simulink model "Ecotron"  (R2019b)
settings: Solver=FixedStepAuto  StartTime=0.0  StopTime=1  FixedStep=0.001  RelTol=1e-3  EnableMultiTasking=on
InitFcn:
  | EcoCoder_PreCheckLic();
libraries: CoderSF_BSW_Libs x228, SF_CanService_Libs x49, simulink x33, dspstat3 x6
(part 3 of 6)

== system Ecotron/Input/PC/FrontWheelCommands ==
  Bus Creator : BusCreator  Inputs=3
  Bus Creator1 : BusCreator  Inputs=4  OutDataTypeStr=Bus: Msg
      settings: InheritFromInputs=off
  Read CAN Message : SF_CanService_Libs/Read CAN Message  typeCAN=Connected  channel=CAN_D  mEn=off  msgInfo=LeoDrive_vw_GOLF  msgItermStore=FrontWheelCommands  msgIterm=FrontWheelCommands  valid=on  stale=on  motoBit=off  setSignalName=on  flgCustomMonitorVariableRules=on  defineSignalName=off  prefixSignal='PC_'  flgValTest=off  flgNoFixed=on  tSample=Task_L1ms  modeCode=Parameterless
  Subsystem1 : Subsystem
  Write and Read Measurement : CoderSF_BSW_Libs/Calibration & Measurement/Write and Read Measurement  variable_name=PC_SetFrontWheelAngle  variable_value=0  variable_type=single  numD=1  unitStr=""  descStr=""
      settings: AttributesFormatString=type:%<variable_type> Dimensions:%<numD>  SourceProductName=EcoCoder Blocks
  Write and Read Measurement1 : CoderSF_BSW_Libs/Calibration & Measurement/Write and Read Measurement  variable_name=PC_SetFrontWheelAngel_Rate  variable_value=0  variable_type=single  numD=1  unitStr=""  descStr=""
      settings: AttributesFormatString=type:%<variable_type> Dimensions:%<numD>  SourceProductName=EcoCoder Blocks
  Out2 : Outport
  wires:
  Read CAN Message/1 -> Subsystem1/1("Available_in ")
  Bus Creator/1 -> Out2/1
  Read CAN Message/4 -> Write and Read Measurement1/1  "PC_setFront_wheel_angle_rate"
  Subsystem1/2(Cnt) -> Bus Creator1/2  "Cnt"
  Read CAN Message/2 -> Subsystem1/2(Msg_cnt)
  Subsystem1/3(Timeout_Err) -> Bus Creator1/3  "Timeout"
  Read CAN Message/3 -> Write and Read Measurement/1  "PC_setFront_wheel_angle"
  Subsystem1/4(Msg_Freq) -> Bus Creator1/4  "MsgFreq"
  Subsystem1/1("Available ") -> Bus Creator1/1  "Available"
  Write and Read Measurement/1 -> Bus Creator/2  "PC_SetFrontWheelAngle"
  Write and Read Measurement1/1 -> Bus Creator/3  "PC_SetFrontWheelAngel_Rate"
  Bus Creator1/1 -> Bus Creator/1  "Msg"

== system Ecotron/Input/PC/LongitudinalCommands ==
  " Override Probe" : CoderSF_BSW_Libs/Calibration & Measurement/ Override Probe  variableName=SetACC  variableValue=0  overrideValue=0  variableDataType=single  variableMin=[]  variableMax=[]  variableUnitStr=""  variableDescStr=""
  Bus Creator : BusCreator  Inputs=3
  Bus Creator1 : BusCreator  Inputs=4  OutDataTypeStr=Bus: Msg
      settings: InheritFromInputs=off
  Read CAN Message : SF_CanService_Libs/Read CAN Message  typeCAN=Connected  channel=CAN_D  mEn=off  msgInfo=LeoDrive_vw_GOLF  msgItermStore=LongitudinalCommandsV1  msgIterm=LongitudinalCommandsV1  valid=on  stale=on  motoBit=off  setSignalName=on  flgCustomMonitorVariableRules=on  defineSignalName=off  prefixSignal='PC_'  flgValTest=off  flgNoFixed=on  tSample=Task_L1ms  modeCode=Parameterless
  Subsystem1 : Subsystem
  Write and Read Measurement : CoderSF_BSW_Libs/Calibration & Measurement/Write and Read Measurement  variable_name=PC_SetLongAcc  variable_value=0  variable_type=single  numD=1  unitStr=""  descStr=""
      settings: AttributesFormatString=type:%<variable_type> Dimensions:%<numD>  SourceProductName=EcoCoder Blocks
  Write and Read Measurement1 : CoderSF_BSW_Libs/Calibration & Measurement/Write and Read Measurement  variable_name=PC_SetLimitVel  variable_value=0  variable_type=single  numD=1  unitStr=""  descStr=""
      settings: AttributesFormatString=type:%<variable_type> Dimensions:%<numD>  SourceProductName=EcoCoder Blocks
  Out2 : Outport
  wires:
  Subsystem1/1("Available ") -> Bus Creator1/1  "Available"
  Subsystem1/4(Msg_Freq) -> Bus Creator1/4  "MsgFreq"
  Subsystem1/3(Timeout_Err) -> Bus Creator1/3  "Timeout"
  Read CAN Message/2 -> Subsystem1/2(Msg_cnt)
  Subsystem1/2(Cnt) -> Bus Creator1/2  "Cnt"
  Read CAN Message/4 -> Write and Read Measurement1/1  "PC_setLimit_velocity"
  Bus Creator/1 -> Out2/1
  Read CAN Message/1 -> Subsystem1/1("Available_in ")
  Read CAN Message/3 -> Write and Read Measurement/1  "PC_setLong_accel"
  Write and Read Measurement/1 -> " Override Probe"/1  "PC_SetLongAcc"
  Write and Read Measurement1/1 -> Bus Creator/3  "PC_SetLimitVel"
  Bus Creator1/1 -> Bus Creator/1  "Msg"
  " Override Probe"/1 -> Bus Creator/2  "SetACCOvrMsr"

== system Ecotron/Input/PC/LongitudinalCommandsV2 ==
  Bus Creator : BusCreator  Inputs=3
  Bus Creator1 : BusCreator  Inputs=4  OutDataTypeStr=Bus: Msg
      settings: InheritFromInputs=off
  Read CAN Message : SF_CanService_Libs/Read CAN Message  typeCAN=Connected  channel=CAN_D  mEn=off  msgInfo=LeoDrive_vw_GOLF  msgItermStore=LongitudinalCommandsV2  msgIterm=LongitudinalCommandsV2  valid=on  stale=on  motoBit=off  setSignalName=on  flgCustomMonitorVariableRules=on  defineSignalName=off  prefixSignal='PC_'  flgValTest=off  flgNoFixed=on  tSample=Task_L1ms  modeCode=Parameterless
  Subsystem1 : Subsystem
  Write and Read Measurement : CoderSF_BSW_Libs/Calibration & Measurement/Write and Read Measurement  variable_name=PC_SetGasPos  variable_value=0  variable_type=single  numD=1  unitStr=""  descStr=""
      settings: AttributesFormatString=type:%<variable_type> Dimensions:%<numD>  SourceProductName=EcoCoder Blocks
  Write and Read Measurement1 : CoderSF_BSW_Libs/Calibration & Measurement/Write and Read Measurement  variable_name=PC_SetBrakePos  variable_value=0  variable_type=single  numD=1  unitStr=""  descStr=""
      settings: AttributesFormatString=type:%<variable_type> Dimensions:%<numD>  SourceProductName=EcoCoder Blocks
  Out2 : Outport
  wires:
  Read CAN Message/1 -> Subsystem1/1("Available_in ")
  Bus Creator/1 -> Out2/1
  Read CAN Message/4 -> Write and Read Measurement1/1  "PC_setBrake_pedal_pos"
  Subsystem1/2(Cnt) -> Bus Creator1/2  "Cnt"
  Read CAN Message/2 -> Subsystem1/2(Msg_cnt)
  Subsystem1/3(Timeout_Err) -> Bus Creator1/3  "Timeout"
  Read CAN Message/3 -> Write and Read Measurement/1  "PC_setGas_pedal_pos"
  Subsystem1/4(Msg_Freq) -> Bus Creator1/4  "MsgFreq"
  Subsystem1/1("Available ") -> Bus Creator1/1  "Available"
  Write and Read Measurement/1 -> Bus Creator/2  "PC_SetGasPos"
  Write and Read Measurement1/1 -> Bus Creator/3  "PC_SetBrakePos"
  Bus Creator1/1 -> Bus Creator/1  "Msg"

== system Ecotron/Input/PC/Vehicle_Commands ==
  Bus Creator : BusCreator  Inputs=8
  Bus Creator1 : BusCreator  Inputs=4  OutDataTypeStr=Bus: Msg
      settings: InheritFromInputs=off
  Read CAN Message : SF_CanService_Libs/Read CAN Message  typeCAN=Connected  channel=CAN_D  mEn=off  msgInfo=LeoDrive_vw_GOLF  msgItermStore=VehicleCommands  msgIterm=VehicleCommands  valid=on  stale=on  motoBit=off  setSignalName=on  flgCustomMonitorVariableRules=on  defineSignalName=off  prefixSignal='PC_'  flgValTest=off  flgNoFixed=on  tSample=Task_L1ms  modeCode=Parameterless
  Subsystem1 : Subsystem
  Terminator1 : Terminator
  Write and Read Measurement : CoderSF_BSW_Libs/Calibration & Measurement/Write and Read Measurement  variable_name=PC_blinker  variable_value=0  variable_type=uint8  numD=1  unitStr=""  descStr=""
      settings: AttributesFormatString=type:%<variable_type> Dimensions:%<numD>  SourceProductName=EcoCoder Blocks
  Write and Read Measurement1 : CoderSF_BSW_Libs/Calibration & Measurement/Write and Read Measurement  variable_name=PC_headlight  variable_value=0  variable_type=uint8  numD=1  unitStr=""  descStr=""
      settings: AttributesFormatString=type:%<variable_type> Dimensions:%<numD>  SourceProductName=EcoCoder Blocks
  Write and Read Measurement2 : CoderSF_BSW_Libs/Calibration & Measurement/Write and Read Measurement  variable_name=PC_wiper  variable_value=0  variable_type=uint8  numD=1  unitStr=""  descStr=""
      settings: AttributesFormatString=type:%<variable_type> Dimensions:%<numD>  SourceProductName=EcoCoder Blocks
  Write and Read Measurement3 : CoderSF_BSW_Libs/Calibration & Measurement/Write and Read Measurement  variable_name=PC_gear  variable_value=0  variable_type=uint8  numD=1  unitStr=""  descStr=""
      settings: AttributesFormatString=type:%<variable_type> Dimensions:%<numD>  SourceProductName=EcoCoder Blocks
  Write and Read Measurement4 : CoderSF_BSW_Libs/Calibration & Measurement/Write and Read Measurement  variable_name=PC_mode  variable_value=0  variable_type=uint8  numD=1  unitStr=""  descStr=""
      settings: AttributesFormatString=type:%<variable_type> Dimensions:%<numD>  SourceProductName=EcoCoder Blocks
  Write and Read Measurement5 : CoderSF_BSW_Libs/Calibration & Measurement/Write and Read Measurement  variable_name=PC_handBrake  variable_value=0  variable_type=uint8  numD=1  unitStr=""  descStr=""
      settings: AttributesFormatString=type:%<variable_type> Dimensions:%<numD>  SourceProductName=EcoCoder Blocks
  Write and Read Measurement6 : CoderSF_BSW_Libs/Calibration & Measurement/Write and Read Measurement  variable_name=PC_LongMode  variable_value=0  variable_type=uint8  numD=1  unitStr=""  descStr=""
      settings: AttributesFormatString=type:%<variable_type> Dimensions:%<numD>  SourceProductName=EcoCoder Blocks
  Out1 : Outport
  wires:
  Subsystem1/2(Cnt) -> Bus Creator1/2  "Cnt"
  Read CAN Message/2 -> Subsystem1/2(Msg_cnt)
  Subsystem1/4(Msg_Freq) -> Bus Creator1/4  "MsgFreq"
  Read CAN Message/7 -> Write and Read Measurement4/1  "PC_mode"
  Bus Creator/1 -> Out1/1
  Subsystem1/3(Timeout_Err) -> Bus Creator1/3  "Timeout"
  Read CAN Message/8 -> Write and Read Measurement5/1  "PC_handBrake"
  Subsystem1/1("Available ") -> Bus Creator1/1  "Available"
  Read CAN Message/3 -> Write and Read Measurement/1  "PC_blinker"
  Read CAN Message/5 -> Write and Read Measurement2/1  "PC_wiper"
  Read CAN Message/1 -> Subsystem1/1("Available_in ")
  Read CAN Message/4 -> Write and Read Measurement1/1  "PC_headlgiht"
  Read CAN Message/10 -> Write and Read Measurement6/1  "PC_LongMode"
  Read CAN Message/9 -> Terminator1/1  "PC_horn"
  Write and Read Measurement/1 -> Bus Creator/2  "PC_blinker"
  Write and Read Measurement1/1 -> Bus Creator/3  "PC_headlight"
  Write and Read Measurement2/1 -> Bus Creator/4  "PC_wiper"
  Read CAN Message/6 -> Write and Read Measurement3/1  "PC_gear"
  Write and Read Measurement3/1 -> Bus Creator/5  "PC_gear"
  Write and Read Measurement4/1 -> Bus Creator/6  "PC_mode"
  Write and Read Measurement5/1 -> Bus Creator/7  "PC_handBrake"
  Bus Creator1/1 -> Bus Creator/1  "Msg"
  Write and Read Measurement6/1 -> Bus Creator/8  "PC_LongMode"

== system Ecotron/Main /Err Handler/Check Brake Err ==
  In1 : Inport
  Bus Creator : BusCreator  Inputs=2
  Bus Selector : BusSelector  OutputSignals=By-wire.RBF_Brake.EPAS_Msg3.BBW_UnderVoltage,By-wire.RBF_Brake.EPAS_Msg3.BBW_OverCurrent,By-wire.RBF_Brake.EPAS_Msg1.Msg.timeout,By-wire.RBF_Brake.EPAS_Msg2.Msg.timeout,By-wire.RBF_Brake.EPAS_Msg3.Msg.timeout
  OR : Logic  Operator=OR  IconShape=distinctive  AllPortsSameDT=off  OutDataTypeStr=boolean
  OR1 : Logic  Operator=OR  Inputs=3  IconShape=distinctive  AllPortsSameDT=off  OutDataTypeStr=boolean
  Out1 : Outport
  wires:
  In1/1 -> Bus Selector/1
  Bus Selector/1 -> OR/1  "<BBW_UnderVoltage>"
  Bus Selector/2 -> OR/2  "<BBW_OverCurrent>"
  Bus Selector/3 -> OR1/1  "<timeout>"
  Bus Selector/4 -> OR1/2  "<timeout>"
  Bus Selector/5 -> OR1/3  "<timeout>"
  OR/1 -> Bus Creator/1  "Brake_SystemErr"
  OR1/1 -> Bus Creator/2  "Brake_HeartBeatErr"
  Bus Creator/1 -> Out1/1

== system Ecotron/Main /Err Handler/Check EPAS Err ==
  In1 : Inport
  Bus Creator : BusCreator  Inputs=2
  Bus Selector : BusSelector  OutputSignals=By-wire.EPAS.EPAS_Msg3.EPAS_UnderVoltage,By-wire.EPAS.EPAS_Msg3.EPAS_OverCurrent,By-wire.EPAS.EPAS_Msg1.Msg.timeout,By-wire.EPAS.EPAS_Msg2.Msg.timeout,By-wire.EPAS.EPAS_Msg3.Msg.timeout
  OR : Logic  Operator=OR  IconShape=distinctive  AllPortsSameDT=off  OutDataTypeStr=boolean
  OR1 : Logic  Operator=OR  Inputs=3  IconShape=distinctive  AllPortsSameDT=off  OutDataTypeStr=boolean
  Epas_Errors : Outport
  wires:
  In1/1 -> Bus Selector/1
  Bus Selector/1 -> OR/1  "<EPAS_UnderVoltage>"
  Bus Selector/2 -> OR/2  "<EPAS_OverCurrent>"
  OR/1 -> Bus Creator/1  "EPAS_SystemErr"
  Bus Selector/3 -> OR1/1  "<timeout>"
  Bus Selector/4 -> OR1/2  "<timeout>"
  Bus Selector/5 -> OR1/3  "<timeout>"
  OR1/1 -> Bus Creator/2  "EPAS_HeartbeatErr"
  Bus Creator/1 -> Epas_Errors/1

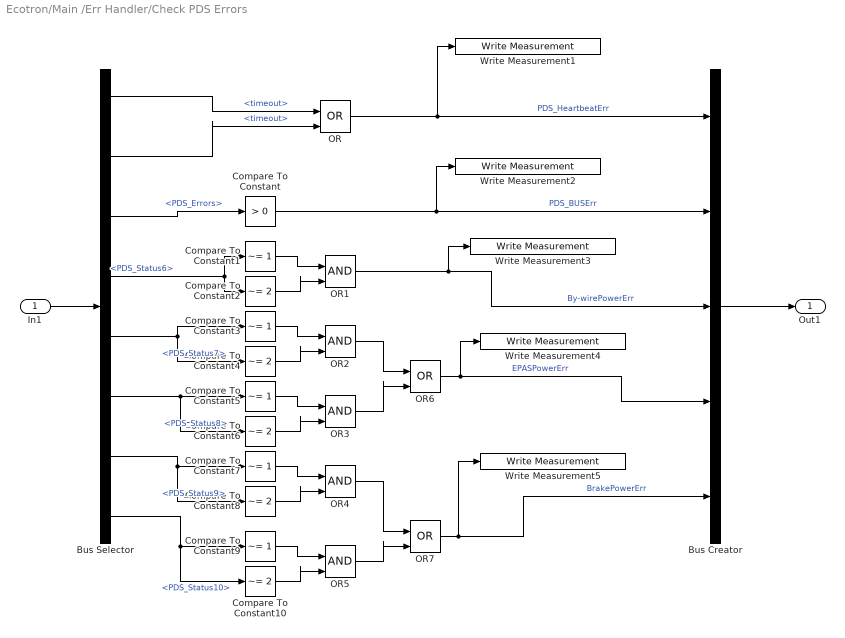
== system Ecotron/Main /Err Handler/Check PDS Errors ==
  In1 : Inport
  Bus Creator : BusCreator  Inputs=5
  Bus Selector : BusSelector  OutputSignals=By-wire.PDS.Status.Msg.timeout,By-wire.PDS.Status2.Msg.timeout,By-wire.PDS.Status.PDS_Errors,By-wire.PDS.Status.PDS_Status6,By-wire.PDS.Status.PDS_Status7,By-wire.PDS.Status.PDS_Status8,By-wire.PDS.Status.PDS_Status9,By-wire.PDS.Status.PDS_Status10
  Compare To Constant : simulink/Logic and Bit Operations/Compare To Constant  relop=>  const=0  OutDataTypeStr=boolean
  Compare To Constant{1,3,5,7,9} (5 alike) : simulink/Logic and Bit Operations/Compare To Constant  relop=~=  const=1  OutDataTypeStr=boolean
  Compare To Constant{2,4,6,8,10} (5 alike) : simulink/Logic and Bit Operations/Compare To Constant  relop=~=  const=2  OutDataTypeStr=boolean
  OR : Logic  Operator=OR  IconShape=distinctive  AllPortsSameDT=off  OutDataTypeStr=boolean
  OR{1..5} (5 alike) : Logic  IconShape=distinctive  AllPortsSameDT=off  OutDataTypeStr=boolean
  OR6 : Logic  Operator=OR  IconShape=distinctive  AllPortsSameDT=off  OutDataTypeStr=boolean
  OR7 : Logic  Operator=OR  IconShape=distinctive  AllPortsSameDT=off  OutDataTypeStr=boolean
  Write Measurement1 : CoderSF_BSW_Libs/Calibration & Measurement/Write Measurement  variable_name=Diag_PDS_HeartbeatErr  variable_value=0  variable_type=boolean  numD=1  unitStr=""  descStr=""
      settings: AttributesFormatString=type:%<variable_type> Dimensions:%<numD>  SourceProductName=EcoCoder Blocks
  Write Measurement2 : CoderSF_BSW_Libs/Calibration & Measurement/Write Measurement  variable_name=Diag_PDS_BUSErr  variable_value=0  variable_type=boolean  numD=1  unitStr=""  descStr=""
      settings: AttributesFormatString=type:%<variable_type> Dimensions:%<numD>  SourceProductName=EcoCoder Blocks
  Write Measurement3 : CoderSF_BSW_Libs/Calibration & Measurement/Write Measurement  variable_name=Diag_By_wirePowerErr  variable_value=0  variable_type=boolean  numD=1  unitStr=""  descStr=""
      settings: AttributesFormatString=type:%<variable_type> Dimensions:%<numD>  SourceProductName=EcoCoder Blocks
  Write Measurement4 : CoderSF_BSW_Libs/Calibration & Measurement/Write Measurement  variable_name=Diag_EPASPowerErr  variable_value=0  variable_type=boolean  numD=1  unitStr=""  descStr=""
      settings: AttributesFormatString=type:%<variable_type> Dimensions:%<numD>  SourceProductName=EcoCoder Blocks
  Write Measurement5 : CoderSF_BSW_Libs/Calibration & Measurement/Write Measurement  variable_name=Diag_BrakePowerErr  variable_value=0  variable_type=boolean  numD=1  unitStr=""  descStr=""
      settings: AttributesFormatString=type:%<variable_type> Dimensions:%<numD>  SourceProductName=EcoCoder Blocks
  Out1 : Outport
  wires:
  In1/1 -> Bus Selector/1
  Bus Selector/1 -> OR/1  "<timeout>"
  Bus Selector/2 -> OR/2  "<timeout>"
  Bus Selector/3 -> Compare To Constant/1  "<PDS_Errors>"
  Bus Selector/4 -> Compare To Constant2/1, Compare To Constant1/1  "<PDS_Status6>"
  Compare To Constant1/1 -> OR1/1
  Compare To Constant2/1 -> OR1/2
  Compare To Constant4/1 -> OR2/2
  Compare To Constant3/1 -> OR2/1
  Compare To Constant5/1 -> OR3/1
  Compare To Constant6/1 -> OR3/2
  Compare To Constant8/1 -> OR4/2
  Compare To Constant7/1 -> OR4/1
  Compare To Constant9/1 -> OR5/1
  Compare To Constant10/1 -> OR5/2
  Bus Selector/5 -> Compare To Constant3/1, Compare To Constant4/1  "<PDS_Status7>"
  Bus Selector/6 -> Compare To Constant6/1, Compare To Constant5/1  "<PDS_Status8>"
  Bus Selector/7 -> Compare To Constant8/1, Compare To Constant7/1  "<PDS_Status9>"
  Bus Selector/8 -> Compare To Constant10/1, Compare To Constant9/1  "<PDS_Status10>"
  OR/1 -> Write Measurement1/1, Bus Creator/1  "PDS_HeartbeatErr"
  Compare To Constant/1 -> Write Measurement2/1, Bus Creator/2  "PDS_BUSErr"
  OR1/1 -> Write Measurement3/1, Bus Creator/3  "By-wirePowerErr"
  OR2/1 -> OR6/1
  OR3/1 -> OR6/2
  OR6/1 -> Write Measurement4/1, Bus Creator/4  "EPASPowerErr"
  OR4/1 -> OR7/1
  OR5/1 -> OR7/2
  OR7/1 -> Write Measurement5/1, Bus Creator/5  "BrakePowerErr"
  Bus Creator/1 -> Out1/1

== system Ecotron/Main /Err Handler/Check Throttle ECU Errors ==
  In1 : Inport
  Bus Creator : BusCreator  Inputs=2
  Bus Selector : BusSelector  OutputSignals=By-wire.Throttle.THROTTLE_CurrentPedalPos,By-wire.Throttle.Msg.timeout
  Compare To Constant : simulink/Logic and Bit Operations/Compare To Constant  relop=>  const=5  OutDataTypeStr=boolean
  Compare To Constant1 : simulink/Logic and Bit Operations/Compare To Constant  relop=>  const=0  OutDataTypeStr=boolean
  Out1 : Outport
  wires:
  In1/1 -> Bus Selector/1
  Bus Selector/1 -> Compare To Constant/1  "<THROTTLE_CurrentPedalPos>"
  Compare To Constant/1 -> Bus Creator/1  "GasPedalintervention"
  Bus Creator/1 -> Out1/1
  Bus Selector/2 -> Compare To Constant1/1  "<timeout>"
  Compare To Constant1/1 -> Bus Creator/2  "Throttle_ECU_HeartbeatErr"

== system Ecotron/Main /Err Handler/MotorStatus ==
  In1 : Inport
  Bus Creator : BusCreator  Inputs=2
  Bus Selector : BusSelector  OutputSignals=vehicle.MotorRotationSpeed.GOLF_MotorRPM,vehicle.Kontak.GOLF_StartStop,vehicle.Kontak.GOLF_KL75
  Compare To Constant : simulink/Logic and Bit Operations/Compare To Constant  relop=>  const=0  OutDataTypeStr=boolean
  Delay : Delay  DelayLength=10  SampleTime=0.1
  OR : Logic  Operator=OR  Inputs=3  IconShape=distinctive  AllPortsSameDT=off  OutDataTypeStr=boolean
  OR1 : Logic  Operator=OR  IconShape=distinctive  AllPortsSameDT=off  OutDataTypeStr=boolean
  RPM : Constant  Value=600  OutDataTypeStr=single
  Relational Operator : RelationalOperator  Operator=<=  OutDataTypeStr=boolean  RndMeth=Simplest
  Write Measurement : CoderSF_BSW_Libs/Calibration & Measurement/Write Measurement  variable_name=Diag_isMotorrunning  variable_value=0  variable_type=boolean  numD=1  unitStr=""  descStr=""
      settings: AttributesFormatString=type:%<variable_type> Dimensions:%<numD>  SourceProductName=EcoCoder Blocks
  Write Measurement1 : CoderSF_BSW_Libs/Calibration & Measurement/Write Measurement  variable_name=Diag_KL75  variable_value=0  variable_type=boolean  numD=1  unitStr=""  descStr=""
      settings: AttributesFormatString=type:%<variable_type> Dimensions:%<numD>  SourceProductName=EcoCoder Blocks
  Motor : Outport
  wires:
  In1/1 -> Bus Selector/1
  Bus Selector/1 -> Relational Operator/2  "<GOLF_MotorRPM>"
  Bus Selector/3 -> Delay/1, OR/2  "<GOLF_KL75>"
  RPM/1 -> Relational Operator/1
  Relational Operator/1 -> OR1/1
  Delay/1 -> OR/3
  OR/1 -> Bus Creator/2, Write Measurement1/1  "Kl75"
  Bus Creator/1 -> Motor/1
  Bus Selector/2 -> Compare To Constant/1  "<GOLF_StartStop>"
  Compare To Constant/1 -> OR1/2
  OR1/1 -> OR/1, Write Measurement/1, Bus Creator/1  "isMotorRunning"

== system Ecotron/Main /Err Handler/Subsystem ==
  In1 : Inport
  AND : Logic  IconShape=distinctive  AllPortsSameDT=off  OutDataTypeStr=boolean
  Bus Selector : BusSelector  OutputSignals=PC.VehicleCMD.Msg.timeout,PC.FrontWheelCMD.Msg.timeout,PC.LongCMD.Msg.timeout,PC.LongV2CMD.Msg.timeout
  OR : Logic  Operator=OR  Inputs=3  IconShape=distinctive  AllPortsSameDT=off  OutDataTypeStr=boolean
  Out1 : Outport
  wires:
  In1/1 -> Bus Selector/1
  Bus Selector/1 -> OR/1  "<timeout>"
  Bus Selector/2 -> OR/2  "<timeout>"
  OR/1 -> Out1/1  "PC_timeout"
  AND/1 -> OR/3
  Bus Selector/3 -> AND/1  "<timeout>"
  Bus Selector/4 -> AND/2  "<timeout>"

== system Ecotron/Main /Gear/Gear_Control ==
  GOLF_CurrentGear : Inport
  Available : Inport  Port=2
  "Set_gear " : Inport  Port=3  OutDataTypeStr=uint8
  Enable : Inport  Port=4
  ParkEnable : Inport  Port=5
  " Override Probe" : CoderSF_BSW_Libs/Calibration & Measurement/ Override Probe  variableName=Set_Gear  variableValue=1  overrideValue=0  variableDataType=uint8  variableMin=[]  variableMax=[]  variableUnitStr=""  variableDescStr=""
      settings: SourceProductName=EcoCoder Blocks
  AND : Logic  IconShape=distinctive  AllPortsSameDT=off  OutDataTypeStr=boolean
  Bus Creator : BusCreator  Inputs=7
  Chart : Stateflow chart  BlockKeywords=__PRM__SERIALIZED__DATA__:Stateflow Chart,Stateflow Diagram  TreatAsAtomicUnit=on
  Chart1 : Stateflow chart  BlockKeywords=__PRM__SERIALIZED__DATA__:Stateflow Chart,Stateflow Diagram  TreatAsAtomicUnit=on
  Data Type Conversion2 : DataTypeConversion  OutDataTypeStr=single
  GOLF_CurrentGear1 : InportShadow
  Read Calibration16 : CoderSF_BSW_Libs/Calibration & Measurement/Read Calibration  variable_name=repeat  variable_value=5  variable_type=single  variable_min=[]  variable_max=[]  unitStr=""  descStr=""
      settings: AttributesFormatString=value:%<variable_value> type:%<variable_type> max:%<variable_max> Min:%<variable_min>  SourceProductName=EcoCoder Blocks
  Read Calibration17 : CoderSF_BSW_Libs/Calibration & Measurement/Read Calibration  variable_name=interval  variable_value=0  variable_type=single  variable_min=[]  variable_max=[]  unitStr=""  descStr=""
      settings: AttributesFormatString=value:%<variable_value> type:%<variable_type> max:%<variable_max> Min:%<variable_min>  SourceProductName=EcoCoder Blocks
  Read Calibration18 : CoderSF_BSW_Libs/Calibration & Measurement/Read Calibration  variable_name=interval2  variable_value=0  variable_type=single  variable_min=[]  variable_max=[]  unitStr=""  descStr=""
      settings: AttributesFormatString=value:%<variable_value> type:%<variable_type> max:%<variable_max> Min:%<variable_min>  SourceProductName=EcoCoder Blocks
  Read Calibration19 : CoderSF_BSW_Libs/Calibration & Measurement/Read Calibration  variable_name=Delay  variable_value=0  variable_type=single  variable_min=[]  variable_max=[]  unitStr=""  descStr=""
      settings: AttributesFormatString=value:%<variable_value> type:%<variable_type> max:%<variable_max> Min:%<variable_min>  SourceProductName=EcoCoder Blocks
  Write Measurement2 : CoderSF_BSW_Libs/Calibration & Measurement/Write Measurement  variable_name=gear_cnt  variable_value=0  variable_type=single  numD=1  unitStr=""  descStr=""
      settings: AttributesFormatString=type:%<variable_type> Dimensions:%<numD>  SourceProductName=EcoCoder Blocks
  Gear_Trigger : Outport
  wires:
  Data Type Conversion2/1 -> Write Measurement2/1
  " Override Probe"/1 -> Chart1/1(SetGear), Chart/2(SetGear)  "Set_GearOvrMsr"
  Available/1 -> Chart1/3(Available)
  Chart1/1(cnt) -> Data Type Conversion2/1
  Read Calibration17/1 -> Chart1/4(interval)
  Read Calibration19/1 -> Chart1/7(delay)
  Read Calibration16/1 -> Chart1/5(msglimit)
  Read Calibration18/1 -> Chart1/6(interval2)
  "Set_gear "/1 -> " Override Probe"/1
  Chart1/2(PtoNTrigger) -> Bus Creator/1  "PtoN"
  Chart1/3(PtoDTrigger) -> Bus Creator/2  "PtoD"
  Chart1/4(DtoNTrigger) -> Bus Creator/3  "DtoN"
  Chart1/5(NtoDTrigger) -> Bus Creator/4  "NtoD"
  Chart1/6(NtoRTrigger) -> Bus Creator/5  "NtoR"
  Chart1/7(RtoNTrigger) -> Bus Creator/6  "RtoN"
  Bus Creator/1 -> Gear_Trigger/1
  Enable/1 -> AND/1, Chart1/8(ENABLE)
  GOLF_CurrentGear/1 -> Chart1/2(CurrentGear)  "GOLF_CurrentGear"
  Chart/1(Parktrigger) -> Bus Creator/7
  GOLF_CurrentGear1/1 -> Chart/1(CurrentGear)  "GOLF_CurrentGear"
  ParkEnable/1 -> AND/2
  AND/1 -> Chart/3(ENABLE)

== system Ecotron/Main /LateralControl/Steering Map ==
  Wheel Rad : Inport
  1-D Lookup Table : Lookup_n-D  NumberOfTableDimensions=1  BreakpointsForDimension1=|  Table=|  InternalRulePriority=Speed  RndMeth=Simplest  InputSameDT=on
      BreakpointsForDimension1=|
      | flip([0.588388039
      | 0.557493058
      | 0.486732906
      | 0.4203094
      | 0.355219971
      | 0.297543446
      | 0.234858963
      | 0.17645621
      | 0.118457225
      | 0.089293954
      | 0.059559667
      | 0.023670812
      | 0.011877895
      | 0.006137322
      | -0.006137322
      | -0.011877895
      | -0.023670812
      | -0.059559667
      | -0.089293954
      | -0.118457225
      | -0.17645621
      | -0.234858963
      | -0.297543446
      | -0.355219971
      | -0.4203094
      | -0.486732906
      | -0.557493058
      | -0.588388039])
      Table=|
      | flip([470
      | 450
      | 400
      | 350
      | 300
      | 250
      | 200
      | 150
      | 100
      | 75
      | 50
      | 20
      | 10
      | 5
      | -5
      | -10
      | -20
      | -50
      | -75
      | -100
      | -150
      | -200
      | -250
      | -300
      | -350
      | -400
      | -450
      | -470
      | ])
  Steering Wheel Degree : Outport
  wires:
  Wheel Rad/1 -> 1-D Lookup Table/1
  1-D Lookup Table/1 -> Steering Wheel Degree/1

== system Ecotron/Main /LongControl /ACC Control ==
  In2 : Inport
  Bus Selector : BusSelector  OutputSignals=input.PC.LongCMD.SetACCOvrMsr,input.vehicle.MotorTorque.GOLF_MotorTorque_filtered,input.vehicle.GearLevel.GOLF_GearLevel,input.vehicle.ACC.GOLF_rxACC
  "Fcalculator " : Subsystem
  Long PID : Subsystem  Commented=on
  StopModeDesicion : Subsystem
  VehicleSpeed : Subsystem
  gas : Outport
  brake : Outport  Port=2
  StopMode : Outport  Port=3
  wires:
  VehicleSpeed/1(m/s) -> StopModeDesicion/1(speed), "Fcalculator "/2(m/s), Long PID/5(speed)
  In2/1 -> Bus Selector/1, "Fcalculator "/1(In1), StopModeDesicion/2(bus), VehicleSpeed/1(In1)
  Bus Selector/1 -> Long PID/1(ACC cmd)  "<SetACCOvrMsr>"
  StopModeDesicion/1(StopModeEnable) -> StopMode/1, "Fcalculator "/3(StopModeEnable), Long PID/6(StopModeEnable)
  Bus Selector/2 -> Long PID/2(MotorTorque)  "<GOLF_MotorTorque_filtered>"
  Bus Selector/3 -> Long PID/3(Gear)  "<GOLF_GearLevel>"
  Bus Selector/4 -> Long PID/4(AccFeedback)  "<GOLF_rxACC>"
  "Fcalculator "/2(Brake Pedal) -> brake/1
  "Fcalculator "/1(Gas Pedal) -> gas/1

== system Ecotron/Main /LongControl /Brake Calib logic ==
  In1 : Inport
  " Override Probe" : CoderSF_BSW_Libs/Calibration & Measurement/ Override Probe  variableName=Brake_CalibCMD  variableValue=0  overrideValue=0  variableDataType=single  variableMin=[]  variableMax=[]  variableUnitStr=""  variableDescStr=""
      settings: SourceProductName=EcoCoder Blocks
  Bus Selector : BusSelector  OutputSignals=Errors.Motor.isMotorRunning,input.vehicle.BrakePedal.GOLF_BrakePedalPos,input.By-wire.RBF_Brake.EPAS_Msg3.BBW_OnCalibration,input.By-wire.RBF_Brake.EPAS_Msg3.BBW_CalibrationErr,input.vehicle.WheelSpeed.GOLF_FLWheelSpeed
  Chart : Stateflow chart  BlockKeywords=__PRM__SERIALIZED__DATA__:Stateflow Chart,Stateflow Diagram  TreatAsAtomicUnit=on
  Out1 : Outport
  wires:
  " Override Probe"/1 -> Out1/1  "Brake_CalibCMDOvrMsr"
  In1/1 -> Bus Selector/1
  Bus Selector/1 -> Chart/1(isMotorRunning)  "<isMotorRunning>"
  Bus Selector/2 -> Chart/2(BrakePedalPos)  "<GOLF_BrakePedalPos>"
  Bus Selector/3 -> Chart/3(BBW_OnCalibration)  "<BBW_OnCalibration>"
  Bus Selector/4 -> Chart/4(BBW_CalibrationErr)  "<BBW_CalibrationErr>"
  Chart/1(Calib_CMD) -> " Override Probe"/1
  Bus Selector/5 -> Chart/5(speed)  "<GOLF_FLWheelSpeed>"

== system Ecotron/Subsystem4/Button cntrl /Subsystem ==
  "Start-Stop " : Inport
  Start_Stop1 : CoderSF_BSW_Libs/Digital I//O/Switch Output  channel=HSO01
      settings: SourceProductName=EcoCoder Blocks
  Start_Stop2 : CoderSF_BSW_Libs/Digital I//O/Switch Output  channel=HSO02
      settings: SourceProductName=EcoCoder Blocks
  Unit Delay : UnitDelay  SampleTime=0.1  HasFrameUpgradeWarning=on
  wires:
  "Start-Stop "/1 -> Start_Stop1/1, Unit Delay/1
  Unit Delay/1 -> Start_Stop2/1

== system Ecotron/Subsystem4/Button cntrl /Subsystem1 ==
  Left_in : Inport
  Right_in : Inport  Port=2
  Hazard_in : Inport  Port=3
  Headligh_in : Inport  Port=4
  Flasher_in : Inport  Port=5
  Mode : Inport  Port=6
  timeout : Inport  Port=7
  AND : Logic  IconShape=distinctive  AllPortsSameDT=off  OutDataTypeStr=boolean
  Compare To Constant : simulink/Logic and Bit Operations/Compare To Constant  relop===  const=1  OutDataTypeStr=boolean
  Compare To Constant1 : simulink/Logic and Bit Operations/Compare To Constant  relop===  const=0  OutDataTypeStr=boolean
  Constant : Constant  Value=0  OutDataTypeStr=boolean
  Switch{,1..4} (5 alike) : Switch  Criteria=u2 > Threshold
  Left_out : Outport
  Right_out : Outport  Port=2
  Hazard_out : Outport  Port=3
  Headlight_out : Outport  Port=4
  Flasher_out : Outport  Port=5
  wires:
  Mode/1 -> Compare To Constant/1
  timeout/1 -> Compare To Constant1/1
  Compare To Constant/1 -> AND/1
  Compare To Constant1/1 -> AND/2
  Left_in/1 -> Switch/1
  Switch/1 -> Left_out/1
  Right_in/1 -> Switch1/1
  Hazard_in/1 -> Switch2/1
  Headligh_in/1 -> Switch3/1
  Flasher_in/1 -> Switch4/1
  AND/1 -> Switch/2, Switch1/2, Switch2/2, Switch3/2, Switch4/2
  Constant/1 -> Switch4/3, Switch3/3, Switch2/3, Switch1/3, Switch/3
  Switch4/1 -> Flasher_out/1
  Switch3/1 -> Headlight_out/1
  Switch2/1 -> Hazard_out/1
  Switch1/1 -> Right_out/1

== system Ecotron/Subsystem4/Button cntrl /Subsystem4 ==
  mode : Inport
  Chart : Stateflow chart  BlockKeywords=__PRM__SERIALIZED__DATA__:Stateflow Chart,Stateflow Diagram  TreatAsAtomicUnit=on
  Falling Edge : CoderSF_BSW_Libs/Application Base Blocks/Falling Edge  InitialCondition=off
      settings: SourceProductName=EcoCoder Blocks
  Read Calibration : CoderSF_BSW_Libs/Calibration & Measurement/Read Calibration  variable_name=Buzz_rising_duration  variable_value=500  variable_type=single  variable_min=[]  variable_max=[]  unitStr=""  descStr=""
      settings: AttributesFormatString=value:%<variable_value> type:%<variable_type> max:%<variable_max> Min:%<variable_min>  SourceProductName=EcoCoder Blocks
  Read Calibration1 : CoderSF_BSW_Libs/Calibration & Measurement/Read Calibration  variable_name=Buzz_falling_duration  variable_value=500  variable_type=single  variable_min=[]  variable_max=[]  unitStr=""  descStr=""
      settings: AttributesFormatString=value:%<variable_value> type:%<variable_type> max:%<variable_max> Min:%<variable_min>  SourceProductName=EcoCoder Blocks
  Read Calibration2 : CoderSF_BSW_Libs/Calibration & Measurement/Read Calibration  variable_name=Buzz_falling_offduration  variable_value=250  variable_type=single  variable_min=[]  variable_max=[]  unitStr=""  descStr=""
      settings: AttributesFormatString=value:%<variable_value> type:%<variable_type> max:%<variable_max> Min:%<variable_min>  SourceProductName=EcoCoder Blocks
  Rising Edge : CoderSF_BSW_Libs/Application Base Blocks/Rising Edge  InitialCondition=on
      settings: SourceProductName=EcoCoder Blocks
  out : Outport
  wires:
  mode/1 -> Falling Edge/1, Rising Edge/1
  Rising Edge/1 -> Chart/1(risingedge)
  Falling Edge/1 -> Chart/2(fallingedge)
  Read Calibration/1 -> Chart/3(rising_duration)
  Read Calibration1/1 -> Chart/4(falling_duration)
  Chart/1(Output) -> out/1
  Read Calibration2/1 -> Chart/5(falling_offduration)

== system Ecotron/Subsystem4/Gear/Drive  ==
  Enable : EnablePort
  Constant : Constant  Value=11
  Constant1 : Constant  Value=9
  Constant2 : Constant
  Constant3 : Constant  Value=150
  Constant4 : Constant  Value=243
  Constant5 : Constant  Value=61
  Constant6 : Constant  Value=82
  Constant7 : Constant  Value=6
  Constant8 : Constant  Value=0
  Send CAN Message 1 : SF_CanService_Libs/Send CAN Message   typeCAN=Connected  channel=CAN_B  mEn=off  msgInfo=vw_golf  msgItermStore=GearShiftSwitch  msgIterm=GearShiftSwitch  motoBit=off  flgNoFixed=on  tSample=Task_Inherit  modeCode=Parameterless  modeRound=Zero
  wires:
  Constant4/1 -> Send CAN Message 1/5
  Constant3/1 -> Send CAN Message 1/4
  Constant8/1 -> Send CAN Message 1/9
  Constant2/1 -> Send CAN Message 1/3
  Constant1/1 -> Send CAN Message 1/2
  Constant7/1 -> Send CAN Message 1/8
  Constant5/1 -> Send CAN Message 1/6
  Constant6/1 -> Send CAN Message 1/7
  Constant/1 -> Send CAN Message 1/1

== system Ecotron/Subsystem4/Gear/Neutral ==
  Enable : EnablePort
  Constant : Constant  Value=53
  Constant1 : Constant  Value=14
  Constant2 : Constant  Value=3
  Constant3 : Constant  Value=150
  Constant4 : Constant  Value=161
  Constant5 : Constant  Value=61
  Constant6 : Constant  Value=82
  Constant7 : Constant  Value=6
  Constant8 : Constant  Value=0
  Send CAN Message 1 : SF_CanService_Libs/Send CAN Message   typeCAN=Connected  channel=CAN_B  mEn=off  msgInfo=vw_golf  msgItermStore=GearShiftSwitch  msgIterm=GearShiftSwitch  motoBit=off  flgNoFixed=on  tSample=Task_MDef  modeCode=Parameterless  modeRound=Zero
  wires:
  Constant/1 -> Send CAN Message 1/1
  Constant6/1 -> Send CAN Message 1/7
  Constant5/1 -> Send CAN Message 1/6
  Constant7/1 -> Send CAN Message 1/8
  Constant1/1 -> Send CAN Message 1/2
  Constant2/1 -> Send CAN Message 1/3
  Constant8/1 -> Send CAN Message 1/9
  Constant3/1 -> Send CAN Message 1/4
  Constant4/1 -> Send CAN Message 1/5

== system Ecotron/Subsystem4/Gear/Reverse ==
  Trigger : TriggerPort  VariantControl=Variant  PortDimensions=1
  Constant : Constant  Value=144
  Constant1 : Constant  Value=10
  Constant2 : Constant  Value=4
  Constant3 : Constant  Value=105
  Constant4 : Constant  Value=0
  Constant5 : Constant  Value=60
  Constant6 : Constant  Value=98
  Constant7 : Constant  Value=6
  Constant8 : Constant  Value=0
  Send CAN Message 1 : SF_CanService_Libs/Send CAN Message   typeCAN=Connected  channel=CAN_B  mEn=off  msgInfo=vw_golf  msgItermStore=GearShiftSwitch  msgIterm=GearShiftSwitch  motoBit=off  flgNoFixed=on  tSample=Task_Inherit  modeCode=Parameterless  modeRound=Zero
  wires:
  Constant4/1 -> Send CAN Message 1/5
  Constant3/1 -> Send CAN Message 1/4
  Constant8/1 -> Send CAN Message 1/9
  Constant2/1 -> Send CAN Message 1/3
  Constant1/1 -> Send CAN Message 1/2
  Constant7/1 -> Send CAN Message 1/8
  Constant5/1 -> Send CAN Message 1/6
  Constant6/1 -> Send CAN Message 1/7
  Constant/1 -> Send CAN Message 1/1

== system Ecotron/Subsystem4/Gear/Reverse1 ==
  Trigger : TriggerPort  VariantControl=Variant  PortDimensions=1
  Constant : Constant  Value=4
  Constant1 : Constant
  Constant2 : Constant  Value=3
  Constant3 : Constant  Value=105
  Constant4 : Constant  Value=0
  Constant5 : Constant  Value=60
  Constant6 : Constant  Value=114
  Constant7 : Constant  Value=6
  Constant8 : Constant  Value=0
  Send CAN Message 1 : SF_CanService_Libs/Send CAN Message   typeCAN=Connected  channel=CAN_B  mEn=off  msgInfo=vw_golf  msgItermStore=GearShiftSwitch  msgIterm=GearShiftSwitch  motoBit=off  flgNoFixed=on  tSample=Task_Inherit  modeCode=Parameterless  modeRound=Zero
  wires:
  Constant/1 -> Send CAN Message 1/1
  Constant6/1 -> Send CAN Message 1/7
  Constant5/1 -> Send CAN Message 1/6
  Constant7/1 -> Send CAN Message 1/8
  Constant1/1 -> Send CAN Message 1/2
  Constant2/1 -> Send CAN Message 1/3
  Constant8/1 -> Send CAN Message 1/9
  Constant3/1 -> Send CAN Message 1/4
  Constant4/1 -> Send CAN Message 1/5

== system Ecotron/Subsystem4/Gear/Reverse2 ==
  Trigger : TriggerPort  VariantControl=Variant  PortDimensions=1
  Constant : Constant  Value=171
  Constant1 : Constant  Value=0
  Constant2 : Constant  Value=2
  Constant3 : Constant  Value=150
  Constant4 : Constant  Value=63
  Constant5 : Constant  Value=61
  Constant6 : Constant  Value=98
  Constant7 : Constant  Value=6
  Constant8 : Constant  Value=0
  Send CAN Message 1 : SF_CanService_Libs/Send CAN Message   typeCAN=Connected  channel=CAN_B  mEn=off  msgInfo=vw_golf  msgItermStore=GearShiftSwitch  msgIterm=GearShiftSwitch  motoBit=off  flgNoFixed=on  tSample=Task_Inherit  modeCode=Parameterless  modeRound=Zero
  wires:
  Constant4/1 -> Send CAN Message 1/5
  Constant3/1 -> Send CAN Message 1/4
  Constant8/1 -> Send CAN Message 1/9
  Constant2/1 -> Send CAN Message 1/3
  Constant1/1 -> Send CAN Message 1/2
  Constant7/1 -> Send CAN Message 1/8
  Constant5/1 -> Send CAN Message 1/6
  Constant6/1 -> Send CAN Message 1/7
  Constant/1 -> Send CAN Message 1/1

== system Ecotron/Subsystem4/Gear/Reverse3 ==
  Trigger : TriggerPort  VariantControl=Variant  PortDimensions=1
  Constant : Constant  Value=228
  Constant1 : Constant  Value=10
  Constant2 : Constant
  Constant3 : Constant  Value=105
  Constant4 : Constant  Value=0
  Constant5 : Constant  Value=60
  Constant6 : Constant  Value=98
  Constant7 : Constant  Value=6
  Constant8 : Constant  Value=0
  Send CAN Message 1 : SF_CanService_Libs/Send CAN Message   typeCAN=Connected  channel=CAN_B  mEn=off  msgInfo=vw_golf  msgItermStore=GearShiftSwitch  msgIterm=GearShiftSwitch  motoBit=off  flgNoFixed=on  tSample=Task_Inherit  modeCode=Parameterless  modeRound=Zero
  wires:
  Constant6/1 -> Send CAN Message 1/7
  Constant4/1 -> Send CAN Message 1/5
  Constant/1 -> Send CAN Message 1/1
  Constant8/1 -> Send CAN Message 1/9
  Constant7/1 -> Send CAN Message 1/8
  Constant1/1 -> Send CAN Message 1/2
  Constant5/1 -> Send CAN Message 1/6
  Constant2/1 -> Send CAN Message 1/3
  Constant3/1 -> Send CAN Message 1/4

== system Ecotron/Subsystem4/PC/Steering Map reverse ==
  Steering Wheel degree : Inport
  1-D Lookup Table : Lookup_n-D  NumberOfTableDimensions=1  BreakpointsForDimension1=|  Table=|  InternalRulePriority=Speed  RndMeth=Simplest  InputSameDT=on
      BreakpointsForDimension1=|
      | flip([470
      | 450
      | 400
      | 350
      | 300
      | 250
      | 200
      | 150
      | 100
      | 75
      | 50
      | 20
      | 10
      | 5
      | -5
      | -10
      | -20
      | -50
      | -75
      | -100
      | -150
      | -200
      | -250
      | -300
      | -350
      | -400
      | -450
      | -470
      | ])
      Table=|
      | flip([0.588388039
      | 0.557493058
      | 0.486732906
      | 0.4203094
      | 0.355219971
      | 0.297543446
      | 0.234858963
      | 0.17645621
      | 0.118457225
      | 0.089293954
      | 0.059559667
      | 0.023670812
      | 0.011877895
      | 0.006137322
      | -0.006137322
      | -0.011877895
      | -0.023670812
      | -0.059559667
      | -0.089293954
      | -0.118457225
      | -0.17645621
      | -0.234858963
      | -0.297543446
      | -0.355219971
      | -0.4203094
      | -0.486732906
      | -0.557493058
      | -0.588388039])
  Wheel Rad : Outport
  wires:
  Steering Wheel degree/1 -> 1-D Lookup Table/1
  1-D Lookup Table/1 -> Wheel Rad/1

== system Ecotron/Subsystem4/PC/VehicleSpeed ==
  In1 : Inport
  Bus Selector : BusSelector  OutputSignals=input.input.vehicle.WheelSpeed.GOLF_BLWheelSpeed,input.input.vehicle.WheelSpeed.GOLF_BRWheelSpeed
  Multiply : Gain  Gain=0.5
  Multiply1 : Gain  Gain=1/3.6
  Sum : Sum  Inputs=|++
  m/s : Outport
  wires:
  In1/1 -> Bus Selector/1
  Bus Selector/1 -> Sum/1  "<GOLF_BLWheelSpeed>"
  Bus Selector/2 -> Sum/2  "<GOLF_BRWheelSpeed>"
  Sum/1 -> Multiply/1
  Multiply/1 -> Multiply1/1
  Multiply1/1 -> m/s/1

== system Ecotron/Subsystem4/PDS/Subsystem ==
  Channel : Inport
  request : Inport  Port=2
  Trigger : TriggerPort  VariantControl=Variant  PortDimensions=1
  "Send CAN Message " : SF_CanService_Libs/Send CAN Message   typeCAN=Connected  channel=CAN_C  mEn=off  msgInfo=ld_pds  msgItermStore=Relay_Request  msgIterm=Relay_Request  motoBit=off  flgNoFixed=on  tSample=Task_Inherit  modeCode=Parameterless  modeRound=Zero
  wires:
  request/1 -> "Send CAN Message "/2
  Channel/1 -> "Send CAN Message "/1

== system Ecotron/Input/By-wire/PDS/Subsystem ==
  Bus Creator1 : BusCreator  Inputs=4  OutDataTypeStr=Bus: Msg
      settings: InheritFromInputs=off
  Bus Creator6 : BusCreator  Inputs=12
  Read CAN Message : SF_CanService_Libs/Read CAN Message  typeCAN=Connected  channel=CAN_C  mEn=off  msgInfo=ld_pds  msgItermStore=PDS_StatusMaster  msgIterm=PDS_StatusMaster  valid=on  stale=on  motoBit=off  setSignalName=on  flgCustomMonitorVariableRules=on  defineSignalName=off  prefixSignal='rx'  flgValTest=off  flgNoFixed=on  tSample=Task_L1ms  modeCode=Parameterless
  Subsystem4 : Subsystem
  Write and Read Measurement : CoderSF_BSW_Libs/Calibration & Measurement/Write and Read Measurement  variable_name=PDS_Status1  variable_value=0  variable_type=uint8  numD=1  unitStr=""  descStr=""
      settings: AttributesFormatString=type:%<variable_type> Dimensions:%<numD>  SourceProductName=EcoCoder Blocks
  Write and Read Measurement1 : CoderSF_BSW_Libs/Calibration & Measurement/Write and Read Measurement  variable_name=PDS_Status2  variable_value=0  variable_type=uint8  numD=1  unitStr=""  descStr=""
      settings: AttributesFormatString=type:%<variable_type> Dimensions:%<numD>  SourceProductName=EcoCoder Blocks
  Write and Read Measurement10 : CoderSF_BSW_Libs/Calibration & Measurement/Write and Read Measurement  variable_name=PDS_Errors  variable_value=0  variable_type=uint8  numD=1  unitStr=""  descStr=""
      settings: AttributesFormatString=type:%<variable_type> Dimensions:%<numD>  SourceProductName=EcoCoder Blocks
  Write and Read Measurement2 : CoderSF_BSW_Libs/Calibration & Measurement/Write and Read Measurement  variable_name=PDS_Status3  variable_value=0  variable_type=uint8  numD=1  unitStr=""  descStr=""
      settings: AttributesFormatString=type:%<variable_type> Dimensions:%<numD>  SourceProductName=EcoCoder Blocks
  Write and Read Measurement3 : CoderSF_BSW_Libs/Calibration & Measurement/Write and Read Measurement  variable_name=PDS_Status4  variable_value=0  variable_type=uint8  numD=1  unitStr=""  descStr=""
      settings: AttributesFormatString=type:%<variable_type> Dimensions:%<numD>  SourceProductName=EcoCoder Blocks
  Write and Read Measurement4 : CoderSF_BSW_Libs/Calibration & Measurement/Write and Read Measurement  variable_name=PDS_Status5  variable_value=0  variable_type=uint8  numD=1  unitStr=""  descStr=""
      settings: AttributesFormatString=type:%<variable_type> Dimensions:%<numD>  SourceProductName=EcoCoder Blocks
  Write and Read Measurement5 : CoderSF_BSW_Libs/Calibration & Measurement/Write and Read Measurement  variable_name=PDS_Status6  variable_value=0  variable_type=uint8  numD=1  unitStr=""  descStr=""
      settings: AttributesFormatString=type:%<variable_type> Dimensions:%<numD>  SourceProductName=EcoCoder Blocks
  Write and Read Measurement6 : CoderSF_BSW_Libs/Calibration & Measurement/Write and Read Measurement  variable_name=PDS_Status7  variable_value=0  variable_type=uint8  numD=1  unitStr=""  descStr=""
      settings: AttributesFormatString=type:%<variable_type> Dimensions:%<numD>  SourceProductName=EcoCoder Blocks
  Write and Read Measurement7 : CoderSF_BSW_Libs/Calibration & Measurement/Write and Read Measurement  variable_name=PDS_Status8  variable_value=0  variable_type=uint8  numD=1  unitStr=""  descStr=""
      settings: AttributesFormatString=type:%<variable_type> Dimensions:%<numD>  SourceProductName=EcoCoder Blocks
  Write and Read Measurement8 : CoderSF_BSW_Libs/Calibration & Measurement/Write and Read Measurement  variable_name=PDS_Status9  variable_value=0  variable_type=uint8  numD=1  unitStr=""  descStr=""
      settings: AttributesFormatString=type:%<variable_type> Dimensions:%<numD>  SourceProductName=EcoCoder Blocks
  Write and Read Measurement9 : CoderSF_BSW_Libs/Calibration & Measurement/Write and Read Measurement  variable_name=PDS_Status10  variable_value=0  variable_type=uint8  numD=1  unitStr=""  descStr=""
      settings: AttributesFormatString=type:%<variable_type> Dimensions:%<numD>  SourceProductName=EcoCoder Blocks
  Status : Outport
  wires:
  Bus Creator6/1 -> Status/1  "Status"
  Subsystem4/2(Cnt) -> Bus Creator1/2  "Cnt"
  Subsystem4/4(Msg_Freq) -> Bus Creator1/4  "MsgFreq"
  Subsystem4/3(Timeout_Err) -> Bus Creator1/3  "Timeout"
  Read CAN Message/2 -> Subsystem4/2(Msg_cnt)
  Read CAN Message/11 -> Write and Read Measurement8/1  "rxSTATUS9"
  Read CAN Message/6 -> Write and Read Measurement3/1  "rxSTATUS4"
  Read CAN Message/9 -> Write and Read Measurement6/1  "rxSTATUS7"
  Subsystem4/1("Available ") -> Bus Creator1/1  "Available"
  Read CAN Message/8 -> Write and Read Measurement5/1  "rxSTATUS6"
  Read CAN Message/7 -> Write and Read Measurement4/1  "rxSTATUS5"
  Bus Creator1/1 -> Bus Creator6/1  "Msg"
  Read CAN Message/4 -> Write and Read Measurement1/1  "rxSTATUS2"
  Read CAN Message/3 -> Write and Read Measurement/1  "rxSTATUS1"
  Read CAN Message/12 -> Write and Read Measurement9/1  "rxSTATUS10"
  Read CAN Message/5 -> Write and Read Measurement2/1  "rxSTATUS3"
  Read CAN Message/10 -> Write and Read Measurement7/1  "rxSTATUS8"
  Read CAN Message/13 -> Write and Read Measurement10/1  "rxErrors"
  Read CAN Message/1 -> Subsystem4/1("Available_in ")
  Write and Read Measurement/1 -> Bus Creator6/2  "PDS_Status1"
  Write and Read Measurement1/1 -> Bus Creator6/3  "PDS_Status2"
  Write and Read Measurement2/1 -> Bus Creator6/4  "PDS_Status3"
  Write and Read Measurement3/1 -> Bus Creator6/5  "PDS_Status4"
  Write and Read Measurement4/1 -> Bus Creator6/6  "PDS_Status5"
  Write and Read Measurement5/1 -> Bus Creator6/7  "PDS_Status6"
  Write and Read Measurement6/1 -> Bus Creator6/8  "PDS_Status7"
  Write and Read Measurement7/1 -> Bus Creator6/9  "PDS_Status8"
  Write and Read Measurement8/1 -> Bus Creator6/10  "PDS_Status9"
  Write and Read Measurement9/1 -> Bus Creator6/11  "PDS_Status10"
  Write and Read Measurement10/1 -> Bus Creator6/12  "PDS_Errors"

== system Ecotron/Input/By-wire/PDS/Subsystem1 ==
  Bus Creator7 : BusCreator  Inputs=3
  Bus Creator8 : BusCreator  Inputs=4  OutDataTypeStr=Bus: Msg
      settings: InheritFromInputs=off
  Read CAN Message4 : SF_CanService_Libs/Read CAN Message  typeCAN=Connected  channel=CAN_C  mEn=off  msgInfo=ld_pds  msgItermStore=PDS_Current3Master  msgIterm=PDS_Current3Master  valid=on  stale=on  motoBit=off  setSignalName=on  flgCustomMonitorVariableRules=on  defineSignalName=off  prefixSignal='rx'  flgValTest=off  flgNoFixed=on  tSample=Task_L1ms  modeCode=Parameterless
  Subsystem6 : Subsystem
  Write and Read Measurement : CoderSF_BSW_Libs/Calibration & Measurement/Write and Read Measurement  variable_name=PDS_CH9Current  variable_value=0  variable_type=single  numD=1  unitStr=""  descStr=""
      settings: AttributesFormatString=type:%<variable_type> Dimensions:%<numD>  SourceProductName=EcoCoder Blocks
  Write and Read Measurement1 : CoderSF_BSW_Libs/Calibration & Measurement/Write and Read Measurement  variable_name=PDS_CH10Current  variable_value=0  variable_type=single  numD=1  unitStr=""  descStr=""
      settings: AttributesFormatString=type:%<variable_type> Dimensions:%<numD>  SourceProductName=EcoCoder Blocks
  Current3 : Outport
  wires:
  Bus Creator8/1 -> Bus Creator7/1  "Msg"
  Read CAN Message4/3 -> Write and Read Measurement/1  "rxCURRENT9"
  Subsystem6/3(Timeout_Err) -> Bus Creator8/3  "Timeout"
  Subsystem6/1("Available ") -> Bus Creator8/1  "Available"
  Subsystem6/4(Msg_Freq) -> Bus Creator8/4  "Freq"
  Read CAN Message4/4 -> Write and Read Measurement1/1  "rxCURRENT10"
  Read CAN Message4/2 -> Subsystem6/2(Msg_cnt)
  Read CAN Message4/1 -> Subsystem6/1("Available_in ")
  Subsystem6/2(Cnt) -> Bus Creator8/2  "Cnt"
  Bus Creator7/1 -> Current3/1  "Current3"
  Write and Read Measurement/1 -> Bus Creator7/2  "PDS_CH9Current"
  Write and Read Measurement1/1 -> Bus Creator7/3  "PDS_CH10Current"
